simulink model "schmehlTangentRotation_th"  (R2018b)
settings: Solver=VariableStepAuto  StartTime=0.0  StopTime=10.0  RelTol=1e-3
libraries: schmehlTangentRotation_ul x1
settings Model: Creator=jldanie5  LastModifiedBy=jldanie5

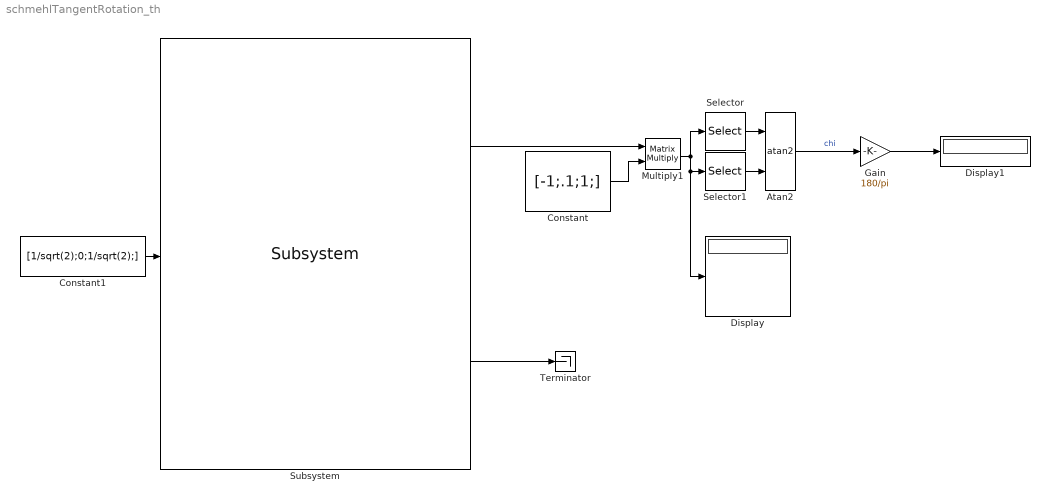
== system schmehlTangentRotation_th ==
  Atan2 : Trigonometry  Operator=atan2
  Constant : Constant  Value=[-1;.1;1;]
  Constant1 : Constant  Value=[1/sqrt(2);0;1/sqrt(2);]
  Display : Display
  Display1 : Display
  Gain : Gain  Gain=180/pi
  Multiply1 : Product  Multiplication=Matrix(*)
  Selector : Selector  InputPortWidth=3  IndexOptions=Index vector (dialog)  Indices=2  OutputSizes=1
  Selector1 : Selector  InputPortWidth=3  IndexOptions=Index vector (dialog)  Indices=1  OutputSizes=1
  Subsystem : schmehlTangentRotation_ul/Subsystem  SystemSampleTime=-1
  Terminator : Terminator
  wires:
  Subsystem/1 -> Multiply1/1
  Subsystem/2 -> Terminator/1
  Constant1/1 -> Subsystem/1
  Constant/1 -> Multiply1/2
  Selector1/1 -> Atan2/2
  Atan2/1 -> Gain/1  "chi"
  Selector/1 -> Atan2/1
  Multiply1/1 -> Display/1, Selector1/1, Selector/1
  Gain/1 -> Display1/1
